simulink model "S6"  (R2016a)
settings: Solver=VariableStepAuto  StartTime=0.0  StopTime=10.0  RelTol=1e-3
settings Model: Creator=asifa  LastModifiedBy=asifa

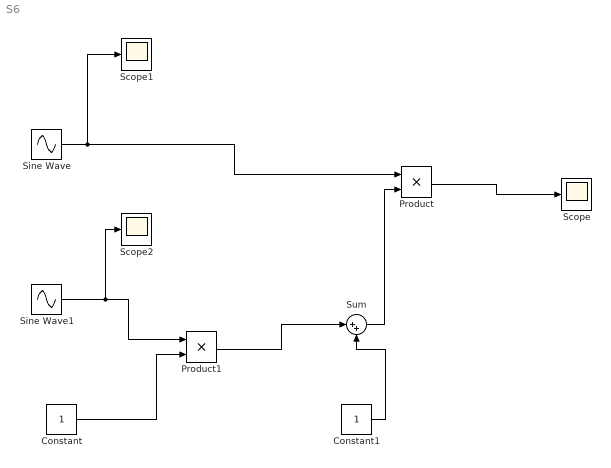
== system S6 ==
  Constant : Constant
  Constant1 : Constant
  Product : Product
  Product1 : Product
  Scope : Scope
  Scope1 : Scope
  Scope2 : Scope
  Sine Wave : Sin  Frequency=2*pi*25  SampleTime=1/5000  VectorParams1D=off
  Sine Wave1 : Sin  Frequency=2*pi  SampleTime=1/5000  VectorParams1D=off
  Sum : Sum  Inputs=|++
  wires:
  Sine Wave1/1 -> Scope2/1, Product1/1
  Constant/1 -> Product1/2
  Sine Wave/1 -> Scope1/1, Product/1
  Product1/1 -> Sum/1
  Constant1/1 -> Sum/2
  Sum/1 -> Product/2
  Product/1 -> Scope/1
